simulink model "pmsm_discrete_variant_closed_loop"  (R2023b)
settings: Solver=FixedStepDiscrete  StartTime=0.0  StopTime=0.1  FixedStep=Ts  RelTol=1e-3
model workspace (MATLAB code in the model file):
  | % Discrete model parameters
  | % Placeholder values for structural execution; no calibration intended.
  | 
  | Ts = 1e-6;              % discrete step [s] (aligned with switching env)
  | 
  | Rs = 0.38;              % PMSM stator resistance [Ohm]   (placeholder)
  | Ld = 1e-3;              % PMSM d-axis inductance [H]     (placeholder)
  | Lq = 1e-3;              % PMSM q-axis inductance [H]     (placeholder)
  | lambda_f = 0.1;         % PMSM flux linkage [Wb]         (placeholder)
libraries: spsControlledCurrentSourceLib x3, spsVoltageMeasurementLib x2, spspowerguiLib x1, spsGroundLib x1, spsSeriesRLCBranchLib x1
settings Model: Creator=hwma  LastModifiedBy=hwma

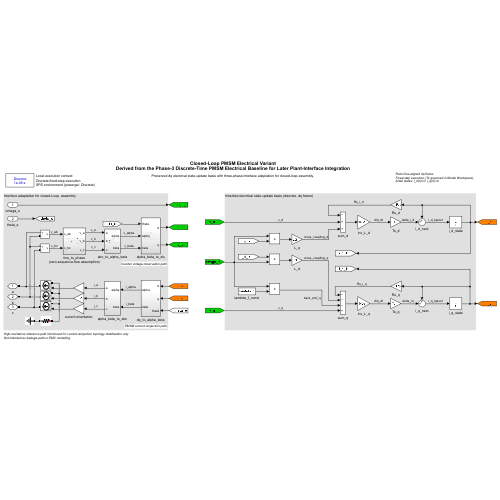
[thumbnail: Simulink's stored preview of the top-level diagram]
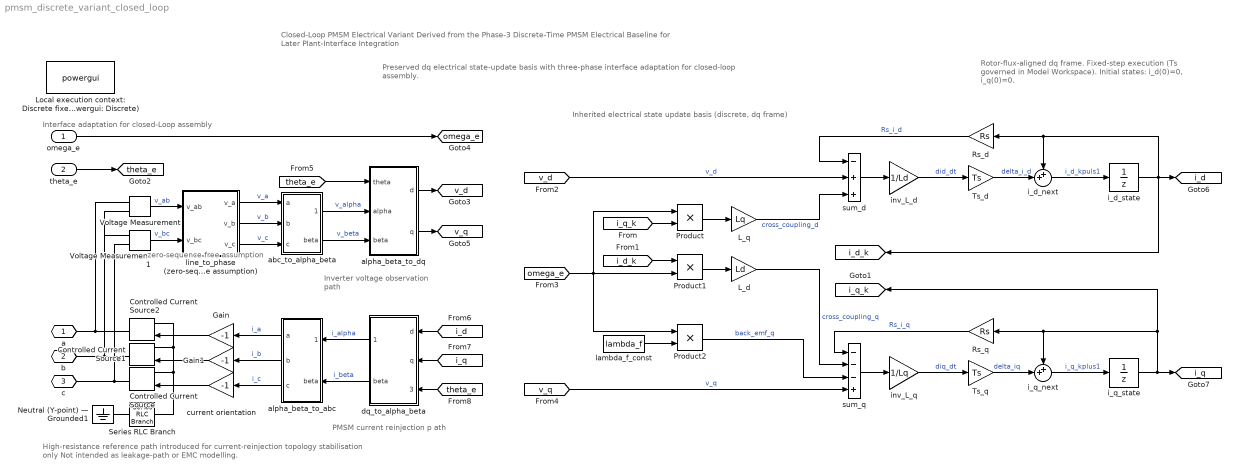
== system pmsm_discrete_variant_closed_loop ==
  note: High-resistance reference path introduced for current-reinjection topology stabilisation only Not intended as leakage-path or EMC modelling.
  note: zero-sequence-free assumption
  note: Inverter voltage observation path
  note: Rotor-flux-aligned dq frame.
      | Fixed-step execution (Ts governed in Model Workspace).
      | Initial states: i_d(0)=0, i_q(0)=0.
  note: Preserved dq electrical state-update basis with three-phase interface adaptation for closed-loop assembly.
  note: Closed-Loop PMSM Electrical Variant
      | Derived from the Phase-3 Discrete-Time PMSM Electrical Baseline for Later Plant-Interface Integration
  note: Inherited electrical state update basis (discrete, dq frame)
  note: Interface adaptation for closed-Loop assembly
  note: PMSM current reinjection p ath
  omega_e : Inport
  theta_e : Inport  Port=2
  Controlled Current Source : spsControlledCurrentSourceLib/Controlled Current Source  Initialize=on  Source_Type=AC  Amplitude=0  Phase=0  Frequency=0  Measurements=None
  Controlled Current Source1 : spsControlledCurrentSourceLib/Controlled Current Source  Initialize=on  Source_Type=AC  Amplitude=0  Phase=0  Frequency=0  Measurements=None
  Controlled Current Source2 : spsControlledCurrentSourceLib/Controlled Current Source  Initialize=on  Source_Type=AC  Amplitude=0  Phase=0  Frequency=0  Measurements=None
  Gain : Gain  Gain=-1
  Gain1 : Gain  Gain=-1
  L_d : Gain  Gain=Ld
  L_q : Gain  Gain=Lq
  Local execution context: Discrete fixed-step execution SPS environment (powergui: Discrete) : spspowerguiLib/powergui  Priority=1  SimulationMode=Discrete  SampleTime=Ts  frequency=60  Iterations=50  frequencyindice=0  Pbase=100e6  ErrMax=1e-4  UnitsV=kV  UnitsW=MW  buscounter=0  FunctionMessages=off  echomessages=off  EnableUseOfTLC=off  CurrentSourceSwitches=off  DisableSnubberDevices=off  DisableRonSwitches=off  DisableVfSwitches=off  DisplayEquations=off  AutomaticDiscreteSolvers=off  SolverType=Tustin/Backward Euler (TBE)  Interpol=off  ExternalGateDelay=off  methode=off  Ts=100  x0status=blocks  SPID=on  SwTol=0  HookPort=off  NonlinearTolerance=1e-4  nMaxIteration=100  ContinueOnMaxIteration=off  RestoreLinks=warning  ResistiveCurrentMeasurement=off  Frange=[0:2:500]  Ylog=off  Xlog=on  ShowGrid=off  save=off  variable=ZData  structure=0  ZoomFFT=off  StartTime=0.0  cycles=1  DisplayStyle=1  fundamental=60  FreqAxis=off  MaxFrequency=1000  frequencyindicesteady=1  RmsSteady=1  display=off
  Neutral (Y-point) — Grounded1 : spsGroundLib/Ground  LConnTagsString=a
  Product : Product
  Product1 : Product
  Product2 : Product
  Rs_d : Gain  Gain=Rs
  Rs_q : Gain  Gain=Rs
  Series RLC Branch : spsSeriesRLCBranchLib/Series RLC Branch  LConnTagsString=__new0  RConnTagsString=__new0  BranchType=R  Resistance=1e7  Inductance=1e-3  SetiL0=off  InitialCurrent=0  Capacitance=1e-3  Setx0=on  InitialVoltage=400  Measurements=None
  Ts_d : Gain  Gain=Ts
  Ts_q : Gain  Gain=Ts
  Voltage Measurement : spsVoltageMeasurementLib/Voltage Measurement  PhasorSimulation=off  OutputType=Complex  PSBequivalent=0
  Voltage Measurement1 : spsVoltageMeasurementLib/Voltage Measurement  PhasorSimulation=off  OutputType=Complex  PSBequivalent=0
  abc_to_alpha_beta : Subsystem
  alpha_beta_to_abc : Subsystem
  alpha_beta_to_dq : Subsystem
  current orientation : Gain  Gain=-1
  dq_to_alpha_beta : Subsystem
  i_d_next : Sum  Inputs=++|
  i_d_state : UnitDelay  SampleTime=Ts  HasFrameUpgradeWarning=on
  i_q_next : Sum  Inputs=++|
  i_q_state : UnitDelay  SampleTime=Ts  HasFrameUpgradeWarning=on
  inv_L_d : Gain  Gain=1/Ld
  inv_L_q : Gain  Gain=1/Lq
  lambda_f_const : Constant  Value=lambda_f
  line_to_phase (zero-sequence-free assumption) : Subsystem
  sum_d : Sum  Inputs=-++
  sum_q : Sum  Inputs=---+
  a : PMIOPort  Side=Left
  b : PMIOPort  Port=2  Side=Left
  c : PMIOPort  Port=3  Side=Left
  tag scope: i_d=global, i_d_k=global, i_q=global, i_q_k=global, omega_e=global, theta_e=global, v_d=global, v_q=global
  wires:
  [v_d] -> sum_d/2  "v_d"
  [v_q] -> sum_q/4  "v_q"
  i_d_state/1 -> [i_d], [i_d_k], i_d_next/1, Rs_d/1
  Rs_d/1 -> sum_d/1  "Rs_i_d"
  Product/1 -> L_q/1
  L_q/1 -> sum_d/3  "cross_coupling_d"
  sum_d/1 -> inv_L_d/1
  inv_L_d/1 -> Ts_d/1  "did_dt"
  i_d_next/1 -> i_d_state/1  "i_d_kpuls1"
  inv_L_q/1 -> Ts_q/1  "diq_dt"
  i_q_state/1 -> [i_q], [i_q_k], Rs_q/1, i_q_next/1
  L_d/1 -> sum_q/2  "cross_coupling_q"
  Product1/1 -> L_d/1
  [omega_e] -> Product2/1, Product1/2, Product/1
  sum_q/1 -> inv_L_q/1
  Rs_q/1 -> sum_q/1  "Rs_i_q"
  Ts_d/1 -> i_d_next/2  "delta_i_d"
  Ts_q/1 -> i_q_next/2  "delta_iq"
  i_q_next/1 -> i_q_state/1  "i_q_kplus1"
  lambda_f_const/1 -> Product2/2
  Product2/1 -> sum_q/3  "back_emf_q"
  [i_q_k] -> Product/2
  [i_d_k] -> Product1/1
  Voltage Measurement/1 -> line_to_phase (zero-sequence-free assumption)/1(v_ab)  "v_ab"
  Voltage Measurement1/1 -> line_to_phase (zero-sequence-free assumption)/2(v_bc)  "v_bc"
  line_to_phase (zero-sequence-free assumption)/1(v_a) -> abc_to_alpha_beta/1(a)  "v_a"
  line_to_phase (zero-sequence-free assumption)/2(v_b) -> abc_to_alpha_beta/2(b)  "v_b"
  line_to_phase (zero-sequence-free assumption)/3(v_c) -> abc_to_alpha_beta/3(c)  "v_c"
  abc_to_alpha_beta/1(alpha) -> alpha_beta_to_dq/2(alpha)  "v_alpha"
  abc_to_alpha_beta/2(beta) -> alpha_beta_to_dq/3(beta)  "v_beta"
  omega_e/1 -> [omega_e]
  theta_e/1 -> [theta_e]
  alpha_beta_to_dq/1(d) -> [v_d]
  alpha_beta_to_dq/2(q) -> [v_q]
  [i_q] -> dq_to_alpha_beta/2(q)
  [i_d] -> dq_to_alpha_beta/1(d)
  [theta_e] -> alpha_beta_to_dq/1(theta)
  [theta_e] -> dq_to_alpha_beta/3(theta)
  dq_to_alpha_beta/2(beta) -> alpha_beta_to_abc/2(beta)  "i_beta"
  dq_to_alpha_beta/1(alpha) -> alpha_beta_to_abc/1(alpha)  "i_alpha"
  alpha_beta_to_abc/1(a) -> Gain/1  "i_a"
  alpha_beta_to_abc/2(b) -> Gain1/1  "i_b"
  alpha_beta_to_abc/3(c) -> current orientation/1  "i_c"
  Gain/1 -> Controlled Current Source2/1
  Gain1/1 -> Controlled Current Source1/1
  current orientation/1 -> Controlled Current Source/1
  connections:
  Voltage Measurement/LConn1 -- Controlled Current Source2/RConn1 -- a/RConn1
  Voltage Measurement/LConn2 -- Voltage Measurement1/LConn1 -- Controlled Current Source1/RConn1 -- b/RConn1
  Voltage Measurement1/LConn2 -- Controlled Current Source/RConn1 -- c/RConn1
  Controlled Current Source2/LConn1 -- Controlled Current Source1/LConn1 -- Series RLC Branch/LConn1 -- Controlled Current Source/LConn1
  Series RLC Branch/RConn1 -- Neutral (Y-point) — Grounded1/LConn1

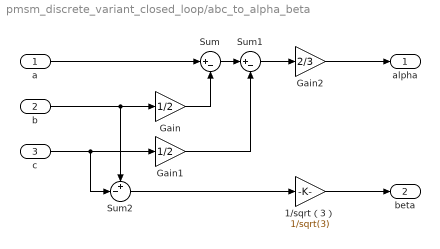
== system pmsm_discrete_variant_closed_loop/abc_to_alpha_beta ==
  a : Inport
  b : Inport  Port=2
  c : Inport  Port=3
  1/sqrt（3） : Gain  Gain=1/sqrt(3)
  Gain : Gain  Gain=1/2
  Gain1 : Gain  Gain=1/2
  Gain2 : Gain  Gain=2/3
  Sum : Sum  Inputs=|+-
  Sum1 : Sum  Inputs=|+-
  Sum2 : Sum  Inputs=+-|
  alpha : Outport
  beta : Outport  Port=2
  wires:
  a/1 -> Sum/1
  b/1 -> Sum2/1, Gain/1
  c/1 -> Sum2/2, Gain1/1
  Gain/1 -> Sum/2
  Sum/1 -> Sum1/1
  Gain1/1 -> Sum1/2
  Sum1/1 -> Gain2/1
  Gain2/1 -> alpha/1
  Sum2/1 -> 1/sqrt（3）/1
  1/sqrt（3）/1 -> beta/1

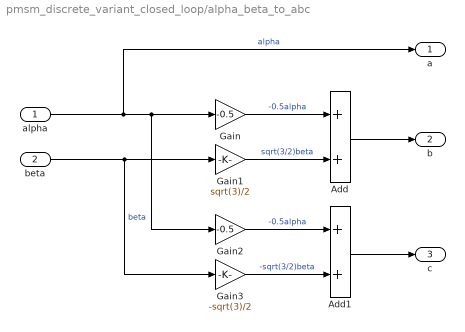
== system pmsm_discrete_variant_closed_loop/alpha_beta_to_abc ==
  alpha : Inport
  beta : Inport  Port=2
  Add : Sum
  Add1 : Sum
  Gain : Gain  Gain=-0.5
  Gain1 : Gain  Gain=sqrt(3)/2
  Gain2 : Gain  Gain=-0.5
  Gain3 : Gain  Gain=-sqrt(3)/2
  a : Outport
  b : Outport  Port=2
  c : Outport  Port=3
  wires:
  beta/1 -> Gain1/1, Gain3/1  "beta"
  Add1/1 -> c/1
  alpha/1 -> a/1, Gain/1, Gain2/1  "alpha"
  Gain3/1 -> Add1/2  "-sqrt(3/2)beta"
  Gain1/1 -> Add/2  "sqrt(3/2)beta"
  Add/1 -> b/1
  Gain2/1 -> Add1/1  "-0.5alpha"
  Gain/1 -> Add/1  "-0.5alpha"

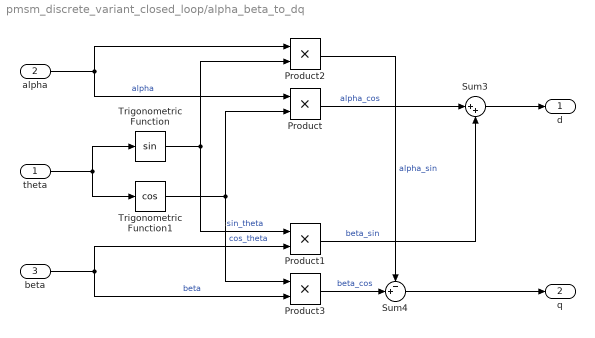
== system pmsm_discrete_variant_closed_loop/alpha_beta_to_dq ==
  theta : Inport
  alpha : Inport  Port=2
  beta : Inport  Port=3
  Product{,1..3} (4 alike) : Product
  Sum3 : Sum  Inputs=|++
  Sum4 : Sum  Inputs=-+|
  Trigonometric Function : Trigonometry
  Trigonometric Function1 : Trigonometry  Operator=cos
  d : Outport
  q : Outport  Port=2
  wires:
  theta/1 -> Trigonometric Function1/1, Trigonometric Function/1
  alpha/1 -> Product2/1, Product/1  "alpha"
  Trigonometric Function1/1 -> Product3/1, Product/2  "cos_theta"
  beta/1 -> Product3/2, Product1/2  "beta"
  Trigonometric Function/1 -> Product2/2, Product1/1  "sin_theta"
  Product/1 -> Sum3/1  "alpha_cos"
  Product1/1 -> Sum3/2  "beta_sin"
  Sum3/1 -> d/1
  Product3/1 -> Sum4/2  "beta_cos"
  Product2/1 -> Sum4/1  "alpha_sin"
  Sum4/1 -> q/1

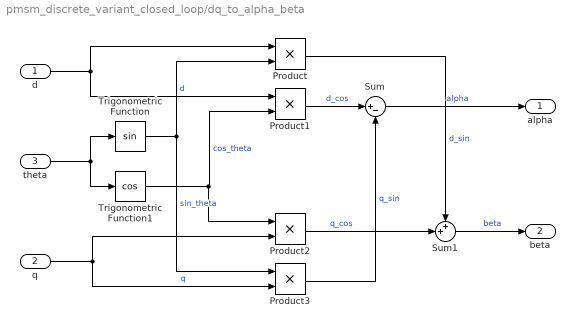
== system pmsm_discrete_variant_closed_loop/dq_to_alpha_beta ==
  d : Inport
  q : Inport  Port=2
  theta : Inport  Port=3
  Product{,1..3} (4 alike) : Product
  Sum : Sum  Inputs=|+-
  Sum1 : Sum  Inputs=++|
  Trigonometric Function : Trigonometry
  Trigonometric Function1 : Trigonometry  Operator=cos
  alpha : Outport
  beta : Outport  Port=2
  wires:
  q/1 -> Product3/2, Product2/2  "q"
  Trigonometric Function1/1 -> Product2/1, Product1/2  "cos_theta"
  Product1/1 -> Sum/1  "d_cos"
  theta/1 -> Trigonometric Function/1, Trigonometric Function1/1
  Trigonometric Function/1 -> Product3/1, Product/2  "sin_theta"
  d/1 -> Product1/1, Product/1  "d"
  Product2/1 -> Sum1/2  "q_cos"
  Product3/1 -> Sum/2  "q_sin"
  Product/1 -> Sum1/1  "d_sin"
  Sum1/1 -> beta/1  "beta"
  Sum/1 -> alpha/1  "alpha"

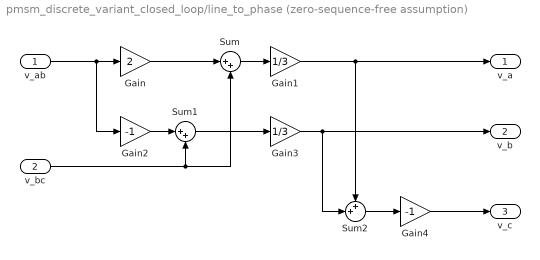
== system pmsm_discrete_variant_closed_loop/line_to_phase (zero-sequence-free assumption) ==
  v_ab : Inport
  v_bc : Inport  Port=2
  Gain : Gain  Gain=2
  Gain1 : Gain  Gain=1/3
  Gain2 : Gain  Gain=-1
  Gain3 : Gain  Gain=1/3
  Gain4 : Gain  Gain=-1
  Sum : Sum  Inputs=|++
  Sum1 : Sum  Inputs=|++
  Sum2 : Sum  Inputs=++|
  v_a : Outport
  v_b : Outport  Port=2
  v_c : Outport  Port=3
  wires:
  v_ab/1 -> Gain2/1, Gain/1
  Gain/1 -> Sum/1
  v_bc/1 -> Sum/2, Sum1/2
  Sum/1 -> Gain1/1
  Gain1/1 -> Sum2/1, v_a/1
  Gain2/1 -> Sum1/1
  Sum1/1 -> Gain3/1
  Gain3/1 -> Sum2/2, v_b/1
  Sum2/1 -> Gain4/1
  Gain4/1 -> v_c/1
